simulink model "SPARCS_Mission_System_Composer"  (R2024a)
settings: Solver=VariableStepAuto  StartTime=0.0  StopTime=10.0  RelTol=1e-3
model workspace (MAT data in the model file):
  Communication_Data_Interface : Simulink.Bus (value not decoded)
  Data_Interface : Simulink.Bus (value not decoded)
  Mechanisem_Interface : Simulink.ConnectionBus (value not decoded)
  Power_Cable : Simulink.ConnectionBus (value not decoded)
  Power_Interface : Simulink.Bus (value not decoded)
undefined symbols (not defined in the file): ADCS, EPS, OBC, Power, TCS, Temp
(part 2 of 2)

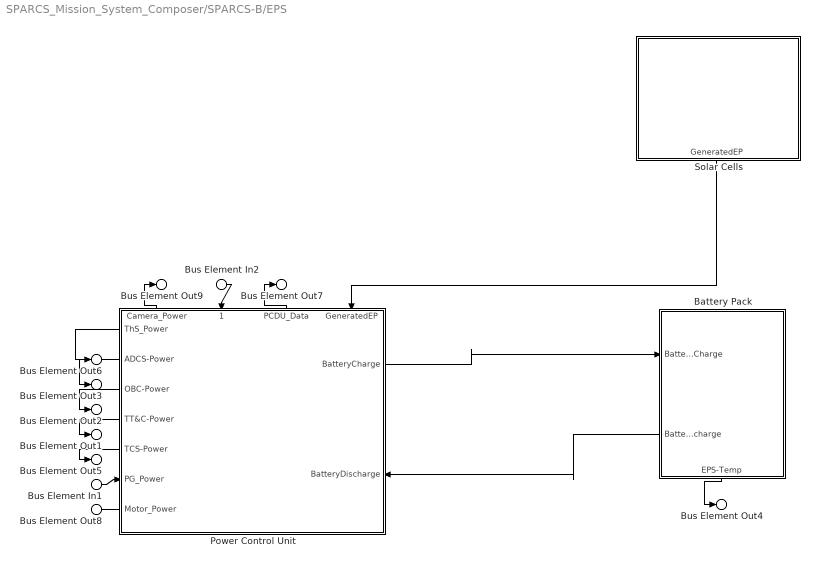
== system SPARCS_Mission_System_Composer/SPARCS-B/EPS ==
  Bus Element In2 : Inport  PortName=EPs_Switch_Command
  Bus Element In1 : Inport  Port=2  PortName=PG_Power
  Battery Pack : Subsystem
      settings: PortSchema="{\"entries\":[{\"content\":{\"headerSize\":26,\"margin\":15,\"minimumSpacing\":25,\"sides\":[{\"content\":{\"connectorIds\":[\"In1\",\"Out2\"]},\"type\":\"ConnectorPlacement.EquallySpacedRectSide\",\"uuid\":\"a0205618-f388-4a93-9aec-aa689e4ebd78\"},{\"content\":{\"connectorIds\":[],\"side\":\"RIGHT\"},\"type\":\"ConnectorPlacement.EquallySpacedRectSide\",\"uuid\":\"79acb52b-c683-45c4-8f19-6aa7b44b6a95\"},{\"content\":{\"connectorIds\":[],\"side\":\"TOP\"},\"type\":\"ConnectorPlacement.EquallySpacedRectSide\",\"uuid\":\"1a3a54da-b4f5-4a0e-9102-49590a789f5c\"},{\"content\":{\"connectorIds\":[\"Out1\"],\"side\":\"BOTTOM\"},\"type\":\"ConnectorPlacement.EquallySpacedRectSide\",\"uuid\":\"779e32a4-6f4c-462e-a89d-e70261c77b0d\"}]},\"type\":\"ConnectorPlacement.EquallySpacedConnector\",\"uuid\":\"e5b731ae-b390-48dd-b7a1-3459e2e6bab0\"}],\"packageUris\":[\"http://schema.mathworks.com/mf0/Connector/R2020b\"],\"version\":\"1.0\"}"
  Power Control Unit : Subsystem
      settings: PortSchema="{\"entries\":[{\"content\":{\"headerSize\":26,\"margin\":15,\"minimumSpacing\":25,\"sides\":[{\"content\":{\"connectorIds\":[\"Out3\",\"Out6\",\"Out8\",\"Out5\",\"Out4\",\"In2\",\"Out7\"]},\"type\":\"ConnectorPlacement.EquallySpacedRectSide\",\"uuid\":\"a0205618-f388-4a93-9aec-aa689e4ebd78\"},{\"content\":{\"connectorIds\":[\"Out9\",\"In4\"],\"side\":\"RIGHT\"},\"type\":\"ConnectorPlacement.EquallySpacedRectSide\",\"uuid\":\"79acb52b-c683-45c4-8f19-6aa7b44b6a95\"},{\"content\":{\"connectorIds\":[\"Out1\",\"In1\",\"Out2\",\"In3\"],\"side\":\"TOP\"},\"type\":\"ConnectorPlacement.EquallySpacedRectSide\",\"uuid\":\"1a3a54da-b4f5-4a0e-9102-49590a789f5c\"},{\"content\":{\"connectorIds\":[],\"side\":\"BOTTOM\"},\"type\":\"ConnectorPlacement.EquallySpacedRectSide\",\"uuid\":\"9b95dc80-80e8-43e3-a13a-4146a26c5b21\"}]},\"type\":\"ConnectorPlacement.EquallySpacedConnector\",\"uuid\":\"e5b731ae-b390-48dd-b7a1-3459e2e6bab0\"}],\"packageUris\":[\"http://schema.mathworks.com/mf0/Connector/R2020b\"],\"version\":\"1.0\"}"
  Solar Cells : Subsystem
      settings: PortSchema="{\"entries\":[{\"content\":{\"headerSize\":26,\"margin\":15,\"minimumSpacing\":25,\"sides\":[{\"content\":{\"connectorIds\":[]},\"type\":\"ConnectorPlacement.EquallySpacedRectSide\",\"uuid\":\"a0205618-f388-4a93-9aec-aa689e4ebd78\"},{\"content\":{\"connectorIds\":[],\"side\":\"RIGHT\"},\"type\":\"ConnectorPlacement.EquallySpacedRectSide\",\"uuid\":\"79acb52b-c683-45c4-8f19-6aa7b44b6a95\"},{\"content\":{\"connectorIds\":[],\"side\":\"TOP\"},\"type\":\"ConnectorPlacement.EquallySpacedRectSide\",\"uuid\":\"1a3a54da-b4f5-4a0e-9102-49590a789f5c\"},{\"content\":{\"connectorIds\":[\"Out1\"],\"side\":\"BOTTOM\"},\"type\":\"ConnectorPlacement.EquallySpacedRectSide\",\"uuid\":\"0fe63fa1-99e2-42a9-86c7-5b07bc6faf14\"}]},\"type\":\"ConnectorPlacement.EquallySpacedConnector\",\"uuid\":\"e5b731ae-b390-48dd-b7a1-3459e2e6bab0\"}],\"packageUris\":[\"http://schema.mathworks.com/mf0/Connector/R2020b\"],\"version\":\"1.0\"}"
  Bus Element Out9 : Outport  PortName=Camera_Power
  Bus Element Out7 : Outport  Port=2  PortName=PCDU_Data
  Bus Element Out8 : Outport  Port=3  PortName=Motor_Power
  Bus Element Out5 : Outport  Port=4  PortName=TCS-Power
  Bus Element Out6 : Outport  Port=5  PortName=ThS_Power
  Bus Element Out4 : Outport  Port=6  PortName=EPS-Temp
  Bus Element Out3 : Outport  Port=7  PortName=ADCS-Power
  Bus Element Out2 : Outport  Port=8  PortName=OBC-Power
  Bus Element Out1 : Outport  Port=9  PortName=TT&C-Power
  wires:
  Battery Pack/2(BatteryDischarge) -> Power Control Unit/4(BatteryDischarge)
  Power Control Unit/9(BatteryCharge) -> Battery Pack/1(BatteryCharge)
  Solar Cells/1(GeneratedEP) -> Power Control Unit/3(GeneratedEP)
  Power Control Unit/6(ADCS-Power) -> Bus Element Out3/1
  Power Control Unit/8(OBC-Power) -> Bus Element Out2/1
  Power Control Unit/5(TT&C-Power) -> Bus Element Out1/1
  Power Control Unit/4(TCS-Power) -> Bus Element Out5/1
  Battery Pack/1(EPS-Temp) -> Bus Element Out4/1
  Bus Element In1/1 -> Power Control Unit/2(PG_Power)
  Power Control Unit/3(ThS_Power) -> Bus Element Out6/1
  Bus Element In2/1 -> Power Control Unit/1(EPs_Switch_Command)
  Power Control Unit/7(Motor_Power) -> Bus Element Out8/1
  Power Control Unit/1(Camera_Power) -> Bus Element Out9/1
  Power Control Unit/2(PCDU_Data) -> Bus Element Out7/1

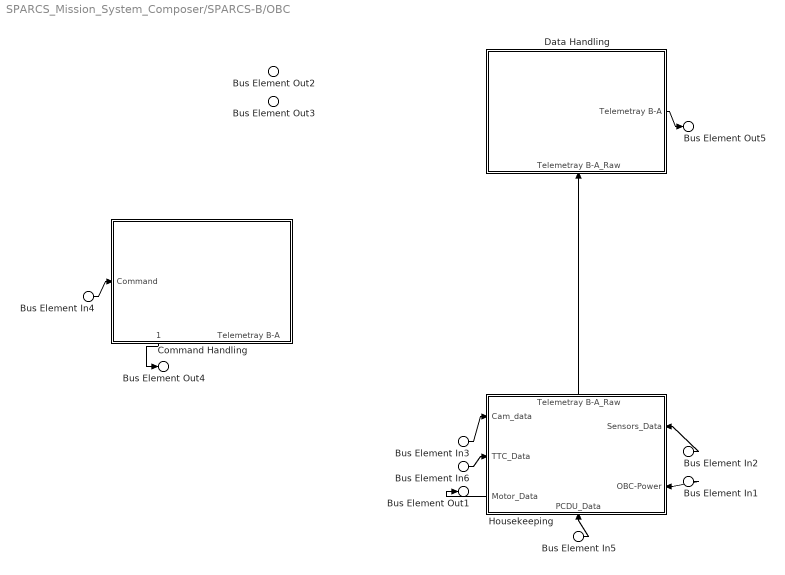
== system SPARCS_Mission_System_Composer/SPARCS-B/OBC ==
  Bus Element In6 : Inport  PortName=TTC_Data
  Bus Element In5 : Inport  Port=2  PortName=PCDU_Data
  Bus Element In4 : Inport  Port=3  PortName=Command
  Bus Element In3 : Inport  Port=4  PortName=Cam_data
  Bus Element In2 : Inport  Port=5  PortName=Sensors_Data
  Bus Element In1 : Inport  Port=6  PortName=OBC-Power
  "Command Handling " : Subsystem
      settings: PortSchema="{\"entries\":[{\"content\":{\"headerSize\":26,\"margin\":15,\"minimumSpacing\":25,\"sides\":[{\"content\":{\"connectorIds\":[\"In2\"]},\"type\":\"ConnectorPlacement.EquallySpacedRectSide\",\"uuid\":\"55446906-0beb-490e-966b-fd119ff7d790\"},{\"content\":{\"connectorIds\":[],\"side\":\"RIGHT\"},\"type\":\"ConnectorPlacement.EquallySpacedRectSide\",\"uuid\":\"4b5c9eb0-c92d-45b7-8098-5a0979f0d9fd\"},{\"content\":{\"connectorIds\":[],\"side\":\"TOP\"},\"type\":\"ConnectorPlacement.EquallySpacedRectSide\",\"uuid\":\"16aec1aa-8dc3-4431-a56b-4fb7824e2a96\"},{\"content\":{\"connectorIds\":[\"Out1\",\"In1\"],\"side\":\"BOTTOM\"},\"type\":\"ConnectorPlacement.EquallySpacedRectSide\",\"uuid\":\"6e384acb-5329-47af-a18c-2030ef64aa13\"}]},\"type\":\"ConnectorPlacement.EquallySpacedConnector\",\"uuid\":\"1865971b-538c-48f2-a7a3-1f3aa40ff883\"}],\"packageUris\":[\"http://schema.mathworks.com/mf0/Connector/R2020b\"],\"version\":\"1.0\"}"
  "Data Handling " : Subsystem
      settings: PortSchema="{\"entries\":[{\"content\":{\"headerSize\":26,\"margin\":15,\"minimumSpacing\":25,\"sides\":[{\"content\":{\"connectorIds\":[]},\"type\":\"ConnectorPlacement.EquallySpacedRectSide\",\"uuid\":\"55446906-0beb-490e-966b-fd119ff7d790\"},{\"content\":{\"connectorIds\":[\"Out1\"],\"side\":\"RIGHT\"},\"type\":\"ConnectorPlacement.EquallySpacedRectSide\",\"uuid\":\"4b5c9eb0-c92d-45b7-8098-5a0979f0d9fd\"},{\"content\":{\"connectorIds\":[],\"side\":\"TOP\"},\"type\":\"ConnectorPlacement.EquallySpacedRectSide\",\"uuid\":\"16aec1aa-8dc3-4431-a56b-4fb7824e2a96\"},{\"content\":{\"connectorIds\":[\"In1\"],\"side\":\"BOTTOM\"},\"type\":\"ConnectorPlacement.EquallySpacedRectSide\",\"uuid\":\"1a5ced55-66af-4bf0-87a3-c6b9f0175afd\"}]},\"type\":\"ConnectorPlacement.EquallySpacedConnector\",\"uuid\":\"1865971b-538c-48f2-a7a3-1f3aa40ff883\"}],\"packageUris\":[\"http://schema.mathworks.com/mf0/Connector/R2020b\"],\"version\":\"1.0\"}"
  Housekeeping : Subsystem
      settings: PortSchema="{\"entries\":[{\"content\":{\"headerSize\":26,\"margin\":15,\"minimumSpacing\":25,\"sides\":[{\"content\":{\"connectorIds\":[\"In3\",\"In4\",\"Out1\"]},\"type\":\"ConnectorPlacement.EquallySpacedRectSide\",\"uuid\":\"55446906-0beb-490e-966b-fd119ff7d790\"},{\"content\":{\"connectorIds\":[\"In1\",\"In2\"],\"side\":\"RIGHT\"},\"type\":\"ConnectorPlacement.EquallySpacedRectSide\",\"uuid\":\"4b5c9eb0-c92d-45b7-8098-5a0979f0d9fd\"},{\"content\":{\"connectorIds\":[\"Out2\"],\"side\":\"TOP\"},\"type\":\"ConnectorPlacement.EquallySpacedRectSide\",\"uuid\":\"16aec1aa-8dc3-4431-a56b-4fb7824e2a96\"},{\"content\":{\"connectorIds\":[\"In5\"],\"side\":\"BOTTOM\"},\"type\":\"ConnectorPlacement.EquallySpacedRectSide\",\"uuid\":\"92354330-e6e6-44e5-aa17-e05d5ad5204a\"}]},\"type\":\"ConnectorPlacement.EquallySpacedConnector\",\"uuid\":\"1865971b-538c-48f2-a7a3-1f3aa40ff883\"}],\"packageUris\":[\"http://schema.mathworks.com/mf0/Connector/R2020b\"],\"version\":\"1.0\"}"
  Bus Element Out3 : Outport  PortName=OutBus
  Bus Element Out2 : Outport  Port=2  PortName=Telemetry B-G
  Bus Element Out5 : Outport  Port=3  PortName=Telemetray B-A
  Bus Element Out4 : Outport  Port=4  PortName=EPs_Switch_Command
  Bus Element Out1 : Outport  Port=5  PortName=Motor_Data
  wires:
  Bus Element In4/1 -> "Command Handling "/2(Command)
  "Command Handling "/1(EPs_Switch_Command) -> Bus Element Out4/1
  Bus Element In5/1 -> Housekeeping/5(PCDU_Data)
  Bus Element In6/1 -> Housekeeping/4(TTC_Data)
  Housekeeping/2(Telemetray B-A_Raw) -> "Data Handling "/1(Telemetray B-A_Raw)
  "Data Handling "/1(Telemetray B-A) -> Bus Element Out5/1
  Bus Element In3/1 -> Housekeeping/3(Cam_data)
  Housekeeping/1(Motor_Data) -> Bus Element Out1/1
  Bus Element In2/1 -> Housekeeping/1(Sensors_Data)
  Bus Element In1/1 -> Housekeeping/2(OBC-Power)

== system SPARCS_Mission_System_Composer/SPARCS-B/TCS ==
  Bus Element In2 : Inport  PortName=EPS-Temp
  Bus Element In1 : Inport  Port=2  PortName=TCS-Power

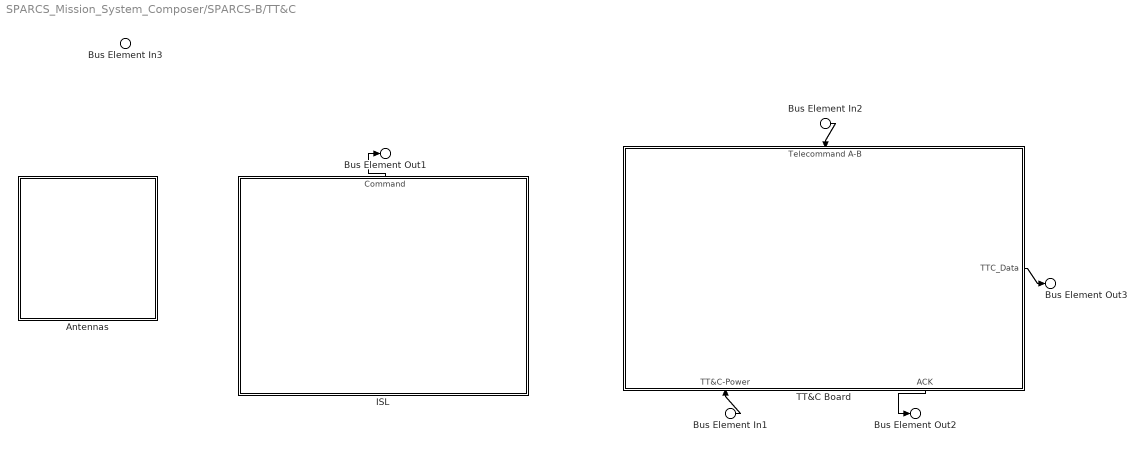
== system SPARCS_Mission_System_Composer/SPARCS-B/TT&C  ==
  Bus Element In3 : Inport  PortName=Telecommand G-B
  Bus Element In2 : Inport  Port=2  PortName=Telecommand A-B
  Bus Element In1 : Inport  Port=3  PortName=TT&C-Power
  Antennas : Subsystem
      settings: PortSchema="{\"entries\":[{\"content\":{\"headerSize\":26,\"margin\":15,\"minimumSpacing\":25,\"sides\":[{\"content\":{\"connectorIds\":[]},\"type\":\"ConnectorPlacement.EquallySpacedRectSide\",\"uuid\":\"b8e64c0e-f241-43e7-badf-308c180049c9\"},{\"content\":{\"connectorIds\":[],\"side\":\"RIGHT\"},\"type\":\"ConnectorPlacement.EquallySpacedRectSide\",\"uuid\":\"146de698-4586-43ed-80a1-9a25d4f72af0\"},{\"content\":{\"connectorIds\":[],\"side\":\"TOP\"},\"type\":\"ConnectorPlacement.EquallySpacedRectSide\",\"uuid\":\"022d51e1-8d8c-4400-9819-a59e0bf78e40\"}]},\"type\":\"ConnectorPlacement.EquallySpacedConnector\",\"uuid\":\"3d3eda84-2dfa-49ef-a4f2-f7a393d07487\"}],\"packageUris\":[\"http://schema.mathworks.com/mf0/Connector/R2020b\"],\"version\":\"1.0\"}"
  ISL : Subsystem
      settings: PortSchema="{\"entries\":[{\"content\":{\"headerSize\":26,\"margin\":15,\"minimumSpacing\":25,\"sides\":[{\"content\":{\"connectorIds\":[]},\"type\":\"ConnectorPlacement.EquallySpacedRectSide\",\"uuid\":\"55446906-0beb-490e-966b-fd119ff7d790\"},{\"content\":{\"connectorIds\":[],\"side\":\"RIGHT\"},\"type\":\"ConnectorPlacement.EquallySpacedRectSide\",\"uuid\":\"4b5c9eb0-c92d-45b7-8098-5a0979f0d9fd\"},{\"content\":{\"connectorIds\":[\"Out1\"],\"side\":\"TOP\"},\"type\":\"ConnectorPlacement.EquallySpacedRectSide\",\"uuid\":\"16aec1aa-8dc3-4431-a56b-4fb7824e2a96\"}]},\"type\":\"ConnectorPlacement.EquallySpacedConnector\",\"uuid\":\"1865971b-538c-48f2-a7a3-1f3aa40ff883\"}],\"packageUris\":[\"http://schema.mathworks.com/mf0/Connector/R2020b\"],\"version\":\"1.0\"}"
  TT&C Board : Subsystem
      settings: PortSchema="{\"entries\":[{\"content\":{\"headerSize\":26,\"margin\":15,\"minimumSpacing\":25,\"sides\":[{\"content\":{\"connectorIds\":[]},\"type\":\"ConnectorPlacement.EquallySpacedRectSide\",\"uuid\":\"b8e64c0e-f241-43e7-badf-308c180049c9\"},{\"content\":{\"connectorIds\":[\"Out1\"],\"side\":\"RIGHT\"},\"type\":\"ConnectorPlacement.EquallySpacedRectSide\",\"uuid\":\"146de698-4586-43ed-80a1-9a25d4f72af0\"},{\"content\":{\"connectorIds\":[\"In2\"],\"side\":\"TOP\"},\"type\":\"ConnectorPlacement.EquallySpacedRectSide\",\"uuid\":\"022d51e1-8d8c-4400-9819-a59e0bf78e40\"},{\"content\":{\"connectorIds\":[\"In1\",\"Out2\"],\"side\":\"BOTTOM\"},\"type\":\"ConnectorPlacement.EquallySpacedRectSide\",\"uuid\":\"5095995b-a4a2-4a84-b5ab-514c2ebaecc0\"}]},\"type\":\"ConnectorPlacement.EquallySpacedConnector\",\"uuid\":\"3d3eda84-2dfa-49ef-a4f2-f7a393d07487\"}],\"packageUris\":[\"http://schema.mathworks.com/mf0/Connector/R2020b\"],\"version\":\"1.0\"}"
  Bus Element Out2 : Outport  PortName=ACK
  Bus Element Out3 : Outport  Port=2  PortName=TTC_Data
  Bus Element Out1 : Outport  Port=3  PortName=Command
  wires:
  Bus Element In2/1 -> TT&C Board/2(Telecommand A-B)
  TT&C Board/2(ACK) -> Bus Element Out2/1
  TT&C Board/1(TTC_Data) -> Bus Element Out3/1
  ISL/1(Command) -> Bus Element Out1/1
  Bus Element In1/1 -> TT&C Board/1(TT&C-Power)

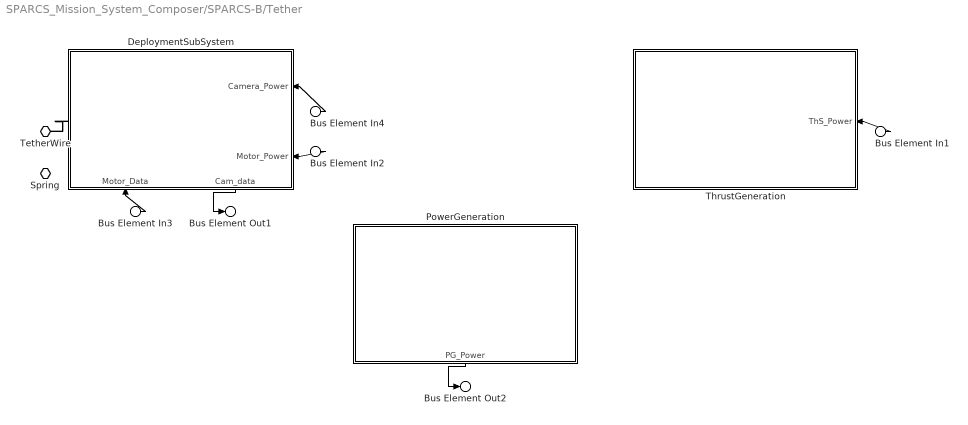
== system SPARCS_Mission_System_Composer/SPARCS-B/Tether ==
  Bus Element In1 : Inport  PortName=ThS_Power
  Bus Element In4 : Inport  Port=2  PortName=Camera_Power
  Bus Element In3 : Inport  Port=3  PortName=Motor_Data
  Bus Element In2 : Inport  Port=4  PortName=Motor_Power
  DeploymentSubSystem : Subsystem
      settings: PortSchema="{\"entries\":[{\"content\":{\"headerSize\":26,\"margin\":15,\"minimumSpacing\":25,\"sides\":[{\"content\":{\"connectorIds\":[\"LConn1\"]},\"type\":\"ConnectorPlacement.EquallySpacedRectSide\",\"uuid\":\"b0f3186e-f576-4647-b1a2-44485358b727\"},{\"content\":{\"connectorIds\":[\"In1\",\"In3\"],\"side\":\"RIGHT\"},\"type\":\"ConnectorPlacement.EquallySpacedRectSide\",\"uuid\":\"71064ded-3aa0-4a06-beed-3d1d2c210288\"},{\"content\":{\"connectorIds\":[],\"side\":\"TOP\"},\"type\":\"ConnectorPlacement.EquallySpacedRectSide\",\"uuid\":\"7b8a25e8-1259-40c4-b5f8-7d1b8fa69d47\"},{\"content\":{\"connectorIds\":[\"In2\",\"Out1\"],\"side\":\"BOTTOM\"},\"type\":\"ConnectorPlacement.EquallySpacedRectSide\",\"uuid\":\"48ecb828-6bd3-4139-bf95-c30462d3ed9f\"}]},\"type\":\"ConnectorPlacement.EquallySpacedConnector\",\"uuid\":\"e60708fb-7212-4361-80b1-30af05aaea9b\"}],\"packageUris\":[\"http://schema.mathworks.com/mf0/Connector/R2020b\"],\"version\":\"1.0\"}"
  PowerGeneration : Subsystem
      settings: PortSchema="{\"entries\":[{\"content\":{\"headerSize\":26,\"margin\":15,\"minimumSpacing\":25,\"sides\":[{\"content\":{\"connectorIds\":[]},\"type\":\"ConnectorPlacement.EquallySpacedRectSide\",\"uuid\":\"b0f3186e-f576-4647-b1a2-44485358b727\"},{\"content\":{\"connectorIds\":[],\"side\":\"RIGHT\"},\"type\":\"ConnectorPlacement.EquallySpacedRectSide\",\"uuid\":\"71064ded-3aa0-4a06-beed-3d1d2c210288\"},{\"content\":{\"connectorIds\":[],\"side\":\"TOP\"},\"type\":\"ConnectorPlacement.EquallySpacedRectSide\",\"uuid\":\"7b8a25e8-1259-40c4-b5f8-7d1b8fa69d47\"},{\"content\":{\"connectorIds\":[\"Out1\"],\"side\":\"BOTTOM\"},\"type\":\"ConnectorPlacement.EquallySpacedRectSide\",\"uuid\":\"bfd9293e-eea8-4d22-ac97-0a750ac877be\"}]},\"type\":\"ConnectorPlacement.EquallySpacedConnector\",\"uuid\":\"e60708fb-7212-4361-80b1-30af05aaea9b\"}],\"packageUris\":[\"http://schema.mathworks.com/mf0/Connector/R2020b\"],\"version\":\"1.0\"}"
  ThrustGeneration : Subsystem
      settings: PortSchema="{\"entries\":[{\"content\":{\"headerSize\":26,\"margin\":15,\"minimumSpacing\":25,\"sides\":[{\"content\":{\"connectorIds\":[]},\"type\":\"ConnectorPlacement.EquallySpacedRectSide\",\"uuid\":\"b0f3186e-f576-4647-b1a2-44485358b727\"},{\"content\":{\"connectorIds\":[\"In1\"],\"side\":\"RIGHT\"},\"type\":\"ConnectorPlacement.EquallySpacedRectSide\",\"uuid\":\"71064ded-3aa0-4a06-beed-3d1d2c210288\"},{\"content\":{\"connectorIds\":[],\"side\":\"TOP\"},\"type\":\"ConnectorPlacement.EquallySpacedRectSide\",\"uuid\":\"7b8a25e8-1259-40c4-b5f8-7d1b8fa69d47\"}]},\"type\":\"ConnectorPlacement.EquallySpacedConnector\",\"uuid\":\"e60708fb-7212-4361-80b1-30af05aaea9b\"}],\"packageUris\":[\"http://schema.mathworks.com/mf0/Connector/R2020b\"],\"version\":\"1.0\"}"
  TetherWire : PMIOPort  Side=Left
  Spring : PMIOPort  Port=2  Side=Left
  Bus Element Out1 : Outport  PortName=Cam_data
  Bus Element Out2 : Outport  Port=2  PortName=PG_Power
  wires:
  DeploymentSubSystem/1(Cam_data) -> Bus Element Out1/1
  Bus Element In2/1 -> DeploymentSubSystem/3(Motor_Power)
  Bus Element In3/1 -> DeploymentSubSystem/2(Motor_Data)
  PowerGeneration/1(PG_Power) -> Bus Element Out2/1
  Bus Element In1/1 -> ThrustGeneration/1(ThS_Power)
  Bus Element In4/1 -> DeploymentSubSystem/1(Camera_Power)
  connections:
  DeploymentSubSystem/LConn1 -- TetherWire/RConn1

== system SPARCS_Mission_System_Composer/Environment/Earth/Magnetic Field ==

== system SPARCS_Mission_System_Composer/Environment/Sun/Sun Vector ==

== system SPARCS_Mission_System_Composer/SPARCS-A/EPS/Battery Pack ==
  Bus Element In1 : Inport  PortName=BatteryCharge
  Bus Element Out2 : Outport  PortName=EPS-Temp
  Bus Element Out1 : Outport  Port=2  PortName=BatteryDischarge

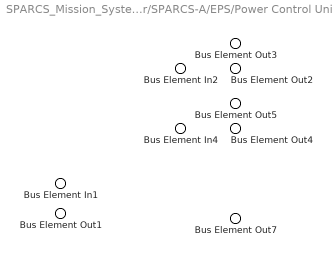
== system SPARCS_Mission_System_Composer/SPARCS-A/EPS/Power Control Unit ==
  Bus Element In4 : Inport  PortName=GeneratedEP
  Bus Element In2 : Inport  Port=2  PortName=EPs_Switch_Command
  Bus Element In1 : Inport  Port=3  PortName=BatteryDischarge
  Bus Element Out5 : Outport  PortName=PCDU_Data
  Bus Element Out3 : Outport  Port=2  PortName=TCS_Power
  Bus Element Out4 : Outport  Port=3  PortName=TT&C_Power
  Bus Element Out7 : Outport  Port=4  PortName=ADCS_Power
  Bus Element Out2 : Outport  Port=5  PortName=OBC_Power
  Bus Element Out1 : Outport  Port=6  PortName=BatteryCharge

== system SPARCS_Mission_System_Composer/SPARCS-A/EPS/SolarCells ==
  Bus Element Out1 : Outport  PortName=GeneratedEP

== system SPARCS_Mission_System_Composer/SPARCS-A/OBC/Command Handling  ==
  Bus Element In1 : Inport  PortName=Command
  Bus Element Out2 : Outport  PortName=Telecommand A-B
  Bus Element Out1 : Outport  Port=2  PortName=EPs_Switch_Command

== system SPARCS_Mission_System_Composer/SPARCS-A/OBC/Data Handling  ==
  Bus Element In2 : Inport  PortName=Telemetray B-A
  Bus Element In1 : Inport  Port=2  PortName=Telemetray B-A_Raw
  Bus Element Out1 : Outport  PortName=Telemetray A-G

== system SPARCS_Mission_System_Composer/SPARCS-A/OBC/Housekeeping ==
  Bus Element In4 : Inport  PortName=Sensors_Data
  Bus Element In5 : Inport  Port=2  PortName=OBC-Power
  Bus Element In2 : Inport  Port=3  PortName=TTC_Data
  Bus Element In1 : Inport  Port=4  PortName=PCDU_Data
  Bus Element Out2 : Outport  PortName=Telemetray B-A_Raw

== system SPARCS_Mission_System_Composer/SPARCS-A/TT&C /Antennas ==

== system SPARCS_Mission_System_Composer/SPARCS-A/TT&C /ISL ==
  Bus Element In1 : Inport  PortName=ACK
  Bus Element Out1 : Outport  PortName=Command

== system SPARCS_Mission_System_Composer/SPARCS-A/TT&C /TT&C Board ==

== system SPARCS_Mission_System_Composer/SPARCS-B/EPS/Battery Pack ==
  Bus Element In1 : Inport  PortName=BatteryCharge
  Bus Element Out2 : Outport  PortName=EPS-Temp
  Bus Element Out1 : Outport  Port=2  PortName=BatteryDischarge

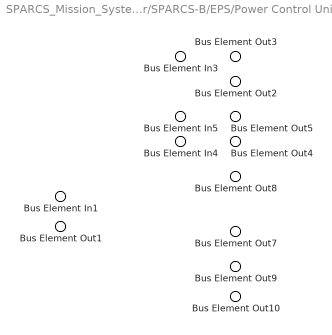
== system SPARCS_Mission_System_Composer/SPARCS-B/EPS/Power Control Unit ==
  Bus Element In5 : Inport  PortName=EPs_Switch_Command
  Bus Element In3 : Inport  Port=2  PortName=PG_Power
  Bus Element In4 : Inport  Port=3  PortName=GeneratedEP
  Bus Element In1 : Inport  Port=4  PortName=BatteryDischarge
  Bus Element Out9 : Outport  PortName=Camera_Power
  Bus Element Out10 : Outport  Port=2  PortName=PCDU_Data
  Bus Element Out5 : Outport  Port=3  PortName=ThS_Power
  Bus Element Out3 : Outport  Port=4  PortName=TCS-Power
  Bus Element Out4 : Outport  Port=5  PortName=TT&C-Power
  Bus Element Out7 : Outport  Port=6  PortName=ADCS-Power
  Bus Element Out8 : Outport  Port=7  PortName=Motor_Power
  Bus Element Out2 : Outport  Port=8  PortName=OBC-Power
  Bus Element Out1 : Outport  Port=9  PortName=BatteryCharge

== system SPARCS_Mission_System_Composer/SPARCS-B/EPS/Solar Cells ==
  Bus Element Out1 : Outport  PortName=GeneratedEP

== system SPARCS_Mission_System_Composer/SPARCS-B/OBC/Command Handling  ==
  Bus Element In2 : Inport  PortName=Telemetray B-A
  Bus Element In1 : Inport  Port=2  PortName=Command
  Bus Element Out1 : Outport  PortName=EPs_Switch_Command

== system SPARCS_Mission_System_Composer/SPARCS-B/OBC/Data Handling  ==
  Bus Element In1 : Inport  PortName=Telemetray B-A_Raw
  Bus Element Out1 : Outport  PortName=Telemetray B-A

== system SPARCS_Mission_System_Composer/SPARCS-B/OBC/Housekeeping ==
  Bus Element In4 : Inport  PortName=Sensors_Data
  Bus Element In5 : Inport  Port=2  PortName=OBC-Power
  Bus Element In3 : Inport  Port=3  PortName=Cam_data
  Bus Element In2 : Inport  Port=4  PortName=TTC_Data
  Bus Element In1 : Inport  Port=5  PortName=PCDU_Data
  Bus Element Out3 : Outport  PortName=Motor_Data
  Bus Element Out2 : Outport  Port=2  PortName=Telemetray B-A_Raw

== system SPARCS_Mission_System_Composer/SPARCS-B/TT&C /Antennas ==

== system SPARCS_Mission_System_Composer/SPARCS-B/TT&C /ISL ==
  Bus Element Out1 : Outport  PortName=Command

== system SPARCS_Mission_System_Composer/SPARCS-B/TT&C /TT&C Board ==
  Bus Element In2 : Inport  PortName=TT&C-Power
  Bus Element In1 : Inport  Port=2  PortName=Telecommand A-B
  Bus Element Out2 : Outport  PortName=TTC_Data
  Bus Element Out1 : Outport  Port=2  PortName=ACK

== system SPARCS_Mission_System_Composer/SPARCS-B/Tether/DeploymentSubSystem ==
  Bus Element In1 : Inport  PortName=Camera_Power
  Bus Element In3 : Inport  Port=2  PortName=Motor_Data
  Bus Element In2 : Inport  Port=3  PortName=Motor_Power
  Camera : Subsystem
      settings: PortSchema="{\"entries\":[{\"content\":{\"headerSize\":26,\"margin\":15,\"minimumSpacing\":25,\"sides\":[{\"content\":{\"connectorIds\":[]},\"type\":\"ConnectorPlacement.EquallySpacedRectSide\",\"uuid\":\"b0f3186e-f576-4647-b1a2-44485358b727\"},{\"content\":{\"connectorIds\":[],\"side\":\"RIGHT\"},\"type\":\"ConnectorPlacement.EquallySpacedRectSide\",\"uuid\":\"71064ded-3aa0-4a06-beed-3d1d2c210288\"},{\"content\":{\"connectorIds\":[\"In1\"],\"side\":\"TOP\"},\"type\":\"ConnectorPlacement.EquallySpacedRectSide\",\"uuid\":\"7b8a25e8-1259-40c4-b5f8-7d1b8fa69d47\"},{\"content\":{\"connectorIds\":[\"Out1\"],\"side\":\"BOTTOM\"},\"type\":\"ConnectorPlacement.EquallySpacedRectSide\",\"uuid\":\"7c86a321-0501-46f7-853d-f0e610ca23c2\"}]},\"type\":\"ConnectorPlacement.EquallySpacedConnector\",\"uuid\":\"e60708fb-7212-4361-80b1-30af05aaea9b\"}],\"packageUris\":[\"http://schema.mathworks.com/mf0/Connector/R2020b\"],\"version\":\"1.0\"}"
  Motor : Subsystem
      settings: PortSchema="{\"entries\":[{\"content\":{\"headerSize\":26,\"margin\":15,\"minimumSpacing\":25,\"sides\":[{\"content\":{\"connectorIds\":[\"LConn1\"]},\"type\":\"ConnectorPlacement.EquallySpacedRectSide\",\"uuid\":\"b0f3186e-f576-4647-b1a2-44485358b727\"},{\"content\":{\"connectorIds\":[],\"side\":\"RIGHT\"},\"type\":\"ConnectorPlacement.EquallySpacedRectSide\",\"uuid\":\"71064ded-3aa0-4a06-beed-3d1d2c210288\"},{\"content\":{\"connectorIds\":[\"In2\"],\"side\":\"TOP\"},\"type\":\"ConnectorPlacement.EquallySpacedRectSide\",\"uuid\":\"7b8a25e8-1259-40c4-b5f8-7d1b8fa69d47\"},{\"content\":{\"connectorIds\":[\"In1\"],\"side\":\"BOTTOM\"},\"type\":\"ConnectorPlacement.EquallySpacedRectSide\",\"uuid\":\"7852af95-d6ff-40f8-9db7-20e88ef59511\"}]},\"type\":\"ConnectorPlacement.EquallySpacedConnector\",\"uuid\":\"e60708fb-7212-4361-80b1-30af05aaea9b\"}],\"packageUris\":[\"http://schema.mathworks.com/mf0/Connector/R2020b\"],\"version\":\"1.0\"}"
  Reel : Subsystem
      settings: PortSchema="{\"entries\":[{\"content\":{\"headerSize\":26,\"margin\":15,\"minimumSpacing\":25,\"sides\":[{\"content\":{\"connectorIds\":[\"LConn1\"]},\"type\":\"ConnectorPlacement.EquallySpacedRectSide\",\"uuid\":\"b0f3186e-f576-4647-b1a2-44485358b727\"},{\"content\":{\"connectorIds\":[\"RConn1\"],\"side\":\"RIGHT\"},\"type\":\"ConnectorPlacement.EquallySpacedRectSide\",\"uuid\":\"71064ded-3aa0-4a06-beed-3d1d2c210288\"},{\"content\":{\"connectorIds\":[],\"side\":\"TOP\"},\"type\":\"ConnectorPlacement.EquallySpacedRectSide\",\"uuid\":\"7b8a25e8-1259-40c4-b5f8-7d1b8fa69d47\"}]},\"type\":\"ConnectorPlacement.EquallySpacedConnector\",\"uuid\":\"e60708fb-7212-4361-80b1-30af05aaea9b\"}],\"packageUris\":[\"http://schema.mathworks.com/mf0/Connector/R2020b\"],\"version\":\"1.0\"}"
  TetherWire : PMIOPort  Side=Left
  Bus Element Out1 : Outport  PortName=Cam_data
  wires:
  Camera/1(Cam_data) -> Bus Element Out1/1
  Bus Element In2/1 -> Motor/2(Motor_Power)
  Bus Element In3/1 -> Motor/1(Motor_Data)
  Bus Element In1/1 -> Camera/1(Camera_Power)
  connections:
  Reel/LConn1 -- TetherWire/RConn1
  Motor/LConn1 -- Reel/RConn1

== system SPARCS_Mission_System_Composer/SPARCS-B/Tether/PowerGeneration ==
  Emitter : Subsystem
      settings: PortSchema="{\"entries\":[{\"content\":{\"headerSize\":26,\"margin\":15,\"minimumSpacing\":25,\"sides\":[{\"content\":{\"connectorIds\":[]},\"type\":\"ConnectorPlacement.EquallySpacedRectSide\",\"uuid\":\"b0f3186e-f576-4647-b1a2-44485358b727\"},{\"content\":{\"connectorIds\":[],\"side\":\"RIGHT\"},\"type\":\"ConnectorPlacement.EquallySpacedRectSide\",\"uuid\":\"71064ded-3aa0-4a06-beed-3d1d2c210288\"},{\"content\":{\"connectorIds\":[],\"side\":\"TOP\"},\"type\":\"ConnectorPlacement.EquallySpacedRectSide\",\"uuid\":\"7b8a25e8-1259-40c4-b5f8-7d1b8fa69d47\"}]},\"type\":\"ConnectorPlacement.EquallySpacedConnector\",\"uuid\":\"e60708fb-7212-4361-80b1-30af05aaea9b\"}],\"packageUris\":[\"http://schema.mathworks.com/mf0/Connector/R2020b\"],\"version\":\"1.0\"}"
  Bus Element Out1 : Outport  PortName=PG_Power

== system SPARCS_Mission_System_Composer/SPARCS-B/Tether/ThrustGeneration ==
  Bus Element In1 : Inport  PortName=ThS_Power
  Collector : Subsystem
      settings: PortSchema="{\"entries\":[{\"content\":{\"headerSize\":26,\"margin\":15,\"minimumSpacing\":25,\"sides\":[{\"content\":{\"connectorIds\":[]},\"type\":\"ConnectorPlacement.EquallySpacedRectSide\",\"uuid\":\"b0f3186e-f576-4647-b1a2-44485358b727\"},{\"content\":{\"connectorIds\":[],\"side\":\"RIGHT\"},\"type\":\"ConnectorPlacement.EquallySpacedRectSide\",\"uuid\":\"71064ded-3aa0-4a06-beed-3d1d2c210288\"},{\"content\":{\"connectorIds\":[],\"side\":\"TOP\"},\"type\":\"ConnectorPlacement.EquallySpacedRectSide\",\"uuid\":\"7b8a25e8-1259-40c4-b5f8-7d1b8fa69d47\"}]},\"type\":\"ConnectorPlacement.EquallySpacedConnector\",\"uuid\":\"e60708fb-7212-4361-80b1-30af05aaea9b\"}],\"packageUris\":[\"http://schema.mathworks.com/mf0/Connector/R2020b\"],\"version\":\"1.0\"}"

== system SPARCS_Mission_System_Composer/SPARCS-B/Tether/DeploymentSubSystem/Camera ==
  Bus Element In1 : Inport  PortName=Camera_Power
  Bus Element Out1 : Outport  PortName=Cam_data

== system SPARCS_Mission_System_Composer/SPARCS-B/Tether/DeploymentSubSystem/Motor ==
  Bus Element In2 : Inport  PortName=Motor_Data
  Bus Element In1 : Inport  Port=2  PortName=Motor_Power
  ReelConn : PMIOPort  Side=Left

== system SPARCS_Mission_System_Composer/SPARCS-B/Tether/DeploymentSubSystem/Reel ==
  TetherWire : PMIOPort  Side=Left
  ReelConn : PMIOPort  Port=2  Side=Right

== system SPARCS_Mission_System_Composer/SPARCS-B/Tether/PowerGeneration/Emitter ==

== system SPARCS_Mission_System_Composer/SPARCS-B/Tether/ThrustGeneration/Collector ==
